simulink model "rls_sim"  (R2017b)
settings: Solver=VariableStepAuto  StartTime=0.0  StopTime=47.1930  RelTol=1e-3
libraries: ctrlSharedLib x2
settings Model: Creator=fortineau_vin  LastModifiedBy=fortineau_vin

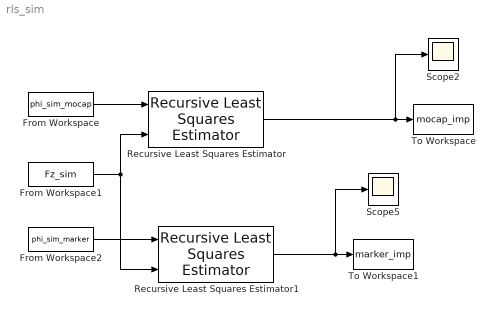
== system rls_sim ==
  From Workspace : FromWorkspace  VariableName=phi_sim_mocap  SampleTime=1e-3
  From Workspace1 : FromWorkspace  VariableName=Fz_sim  SampleTime=1e-3
  From Workspace2 : FromWorkspace  VariableName=phi_sim_marker  SampleTime=1e-3
  Recursive Least Squares Estimator : ctrlSharedLib/Recursive Least Squares Estimator  InitialEstimateSource=None  InitialParameterData=3  P0=1e4  EstimationMethod=Forgetting Factor  AdaptationParameter=0.995  HasTimeVaryingAdaptationParameter=off  NormalizationBias=eps  OutputError=off  OutputP=off  AddEnablePort=off  Ts=-1
      settings: SourceProductName=Control System Toolbox  SourceProductBaseCode=CT
  Recursive Least Squares Estimator1 : ctrlSharedLib/Recursive Least Squares Estimator  InitialEstimateSource=None  InitialParameterData=3  P0=1e4  EstimationMethod=Forgetting Factor  AdaptationParameter=0.995  HasTimeVaryingAdaptationParameter=off  NormalizationBias=eps  OutputError=off  OutputP=off  AddEnablePort=off  Ts=-1
      settings: SourceProductName=Control System Toolbox  SourceProductBaseCode=CT
  Scope2 : Scope
  Scope5 : Scope
  To Workspace : ToWorkspace  VariableName=mocap_imp  SampleTime=-1
  To Workspace1 : ToWorkspace  VariableName=marker_imp  SampleTime=-1
  wires:
  From Workspace/1 -> Recursive Least Squares Estimator/1
  Recursive Least Squares Estimator/1 -> Scope2/1, To Workspace/1
  Recursive Least Squares Estimator1/1 -> To Workspace1/1, Scope5/1
  From Workspace1/1 -> Recursive Least Squares Estimator1/2, Recursive Least Squares Estimator/2
  From Workspace2/1 -> Recursive Least Squares Estimator1/1
